simulink model "Lead_Compensator"  (R2024b)
settings: Solver=VariableStepAuto  StartTime=0.0  StopTime=60  RelTol=1e-3
libraries: cstblocks x4, simulink x1
settings Model: Creator=mafur  LastModifiedBy=mafur

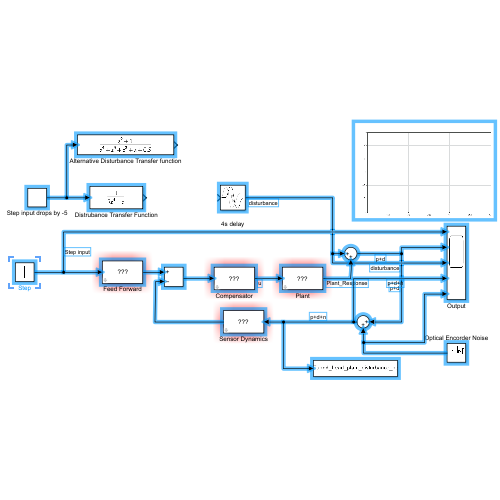
[thumbnail: Simulink's stored preview of the top-level diagram]
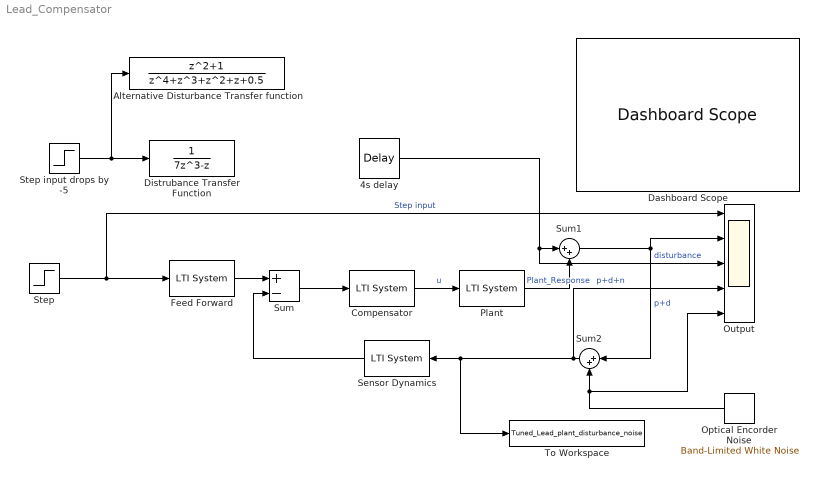
== system Lead_Compensator ==
  " 4s delay" : TransportDelay  DelayTime=40
  Alternative Disturbance Transfer function : DiscreteTransferFcn  Numerator=[1 0 1]  Denominator=[1 1 1 1 0.5]
  Compensator : cstblocks/LTI System  sys=C_Design3  IC=[]  PadeOrder=0
  Dashboard Scope : DashboardScope
  Distrubance Transfer Function : DiscreteTransferFcn  Denominator=[7 0 -1 0]
  Feed Forward : cstblocks/LTI System  sys=F  IC=[]  PadeOrder=0
  Optical Encorder Noise : simulink/Sources/Band-Limited White Noise  Cov=[0.000]  Ts=0.1  seed=[23341]
  Output : Scope  NumInputPorts=5
  Plant : cstblocks/LTI System  sys=G  IC=[]  PadeOrder=0
  Sensor Dynamics : cstblocks/LTI System  sys=H  IC=[]  PadeOrder=0
  Step : Step  After=10  SampleTime=0
  Step input drops by -5 : Step  After=-5  SampleTime=0
  Sum : Sum  Inputs=+-
  Sum1 : Sum  Inputs=|++
  Sum2 : Sum  Inputs=|++
  To Workspace : ToWorkspace  VariableName=Tuned_Lead_plant_disturbance_noise  SaveFormat=Structure With Time  SampleTime=-1
  wires:
  Step/1 -> Output/1, Feed Forward/1  "Step input"
  Compensator/1 -> Plant/1  "u"
  Sum/1 -> Compensator/1
  Sensor Dynamics/1 -> Sum/2
  Optical Encorder Noise/1 -> Output/5, Sum2/2
  Step input drops by -5/1 -> Alternative Disturbance Transfer function/1, Distrubance Transfer Function/1
  Feed Forward/1 -> Sum/1
  " 4s delay"/1 -> Sum1/1, Output/3  "disturbance"
  Plant/1 -> Sum1/2  "Plant_Response"
  Sum1/1 -> Sum2/1, Output/2  "p+d"
  Sum2/1 -> To Workspace/1, Sensor Dynamics/1, Output/4  "p+d+n"
